simulink model "change_monitor"  (R2021a)
settings: configuration reference "motor_ctrl_config" (kept outside this file)
libraries: simulink x6
settings Model: DataDictionary=motor_ctrl_data.sldd  OrderedModelArguments=off  Creator=Litao  LastModifiedBy=Litao
settings ConfigSetRef: SourceName=motor_ctrl_config

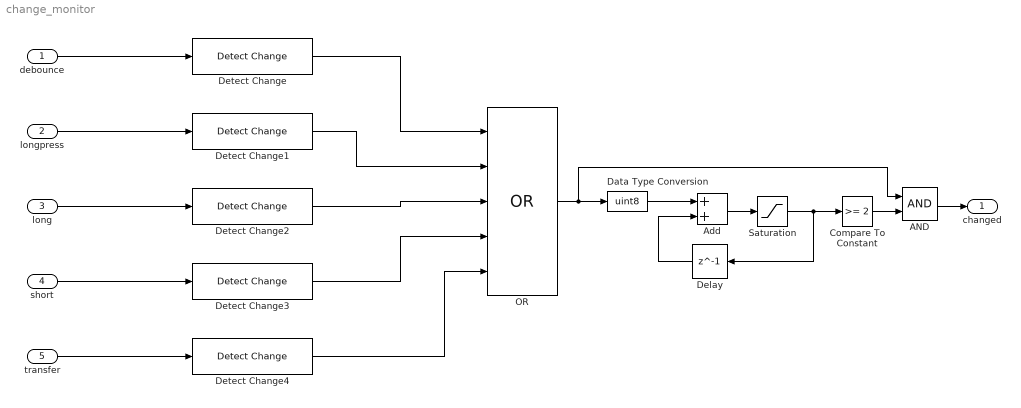
== system change_monitor ==
  debounce : Inport  OutDataTypeStr=int16
  longpress : Inport  Port=2  OutDataTypeStr=int16
  long : Inport  Port=3  OutDataTypeStr=int16
  short : Inport  Port=4  OutDataTypeStr=int16
  transfer : Inport  Port=5  OutDataTypeStr=int16
  AND : Logic  AllPortsSameDT=off  OutDataTypeStr=boolean
  Add : Sum
  Compare To Constant : simulink/Logic and Bit Operations/Compare To Constant  relop=>=  const=2  OutDataTypeStr=boolean
  Data Type Conversion : DataTypeConversion  OutDataTypeStr=uint8
  Delay : Delay  DelayLength=1  InitialCondition=0
  Detect Change{,1..4} (5 alike) : simulink/Logic and Bit Operations/Detect Change  vinit=0  OutDataTypeStr=boolean
  OR : Logic  Operator=OR  Inputs=5  AllPortsSameDT=off  OutDataTypeStr=boolean
  Saturation : Saturate  UpperLimit=100  LowerLimit=0
  changed : Outport
  wires:
  debounce/1 -> Detect Change/1
  longpress/1 -> Detect Change1/1
  long/1 -> Detect Change2/1
  short/1 -> Detect Change3/1
  transfer/1 -> Detect Change4/1
  Detect Change/1 -> OR/1
  Detect Change1/1 -> OR/2
  Detect Change2/1 -> OR/3
  Detect Change3/1 -> OR/4
  Detect Change4/1 -> OR/5
  Add/1 -> Saturation/1
  Compare To Constant/1 -> AND/2
  OR/1 -> Data Type Conversion/1, AND/1
  Data Type Conversion/1 -> Add/1
  AND/1 -> changed/1
  Delay/1 -> Add/2
  Saturation/1 -> Compare To Constant/1, Delay/1
